simulink model "untitled3"  (R2018b)
settings: Solver=VariableStepAuto  StartTime=0.0  StopTime=5  RelTol=1e-3
libraries: commchan3 x1, dsparch4 x1
settings Model: Creator=nhat  LastModifiedBy=nhat

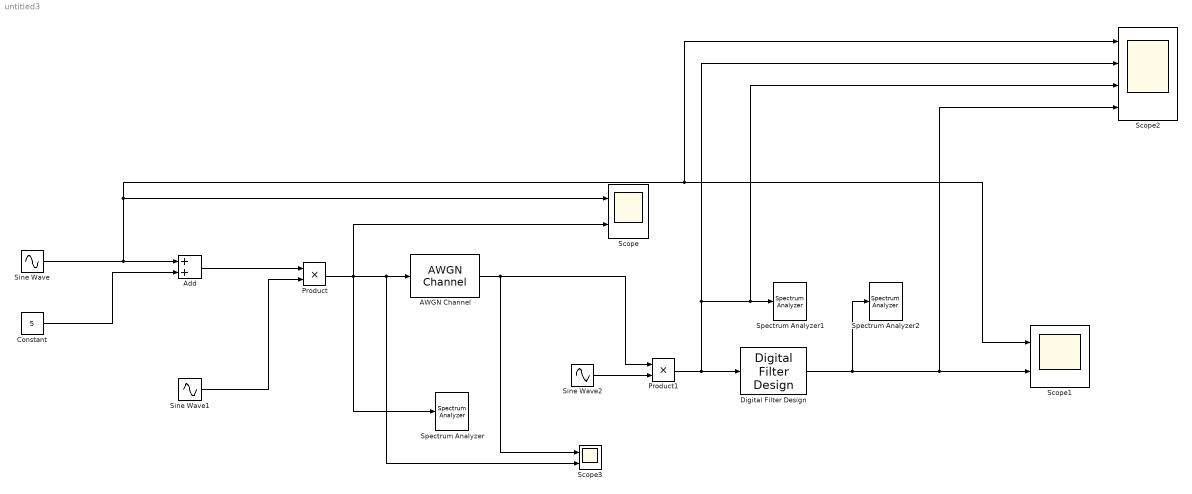
== system untitled3 ==
  AWGN Channel : commchan3/AWGN Channel  InputProcessing=Columns as channels (frame based)  seed=67  noiseMode=Variance from mask  EbNodB=10  EsNodB=10  SNRdB=10  bitsPerSym=1  Ps=1  Tsym=1  variance=1
  Add : Sum
  Constant : Constant  Value=5
  Digital Filter Design : dsparch4/Digital Filter Design  mwdsp_browser_bugfix_var=off
  Product : Product
  Product1 : Product
  Scope : Scope  NumInputPorts=2
  Scope1 : Scope  NumInputPorts=2
  Scope2 : Scope  NumInputPorts=4
  Scope3 : Scope  NumInputPorts=2
  Sine Wave : Sin  Frequency=1000*2*pi  SampleTime=1/100000
  Sine Wave1 : Sin  Frequency=10000*2*pi  SampleTime=1/100000
  Sine Wave2 : Sin  Amplitude=5  Frequency=10000*2*pi  SampleTime=1/100000
  Spectrum Analyzer : SpectrumAnalyzer
  Spectrum Analyzer1 : SpectrumAnalyzer
  Spectrum Analyzer2 : SpectrumAnalyzer
  wires:
  Sine Wave1/1 -> Product/2
  Sine Wave/1 -> Add/1, Scope2/1, Scope1/1, Scope/1
  Product/1 -> Scope/2, AWGN Channel/1, Scope3/2, Spectrum Analyzer/1
  Product1/1 -> Scope2/2, Spectrum Analyzer1/1, Scope2/3, Digital Filter Design/1
  Digital Filter Design/1 -> Scope2/4, Scope1/2, Spectrum Analyzer2/1
  Sine Wave2/1 -> Product1/2
  AWGN Channel/1 -> Product1/1, Scope3/1
  Constant/1 -> Add/2
  Add/1 -> Product/1
